simulink model "dc_servo_HighGainCommand"  (R2020b)
settings: Solver=ode5  StartTime=0.0  StopTime=.25  FixedStep=.00001  RelTol=1e-6  AbsTol=1e-6
values from neighbouring files (symbols this model uses):
  encoder = 2000    [dc_servo_HighGainCommand_data.m]    (also in dc_servo_speed_estimation_data.m)
  f = 4e-4    (= 0.0004)    [dc_servo_HighGainCommand_data.m]    (also in dc_servo_speed_estimation_data.m)
  imax = 5    [dc_servo_HighGainCommand_data.m]    (also in dc_servo_speed_estimation_data.m)
  integrator_saturation = 10000    [dc_servo_HighGainCommand_data.m]    (also in dc_servo_speed_estimation_data.m)
  J = 6.0e-5    (= 6e-05)    [dc_servo_HighGainCommand_data.m]    (also in dc_servo_speed_estimation_data.m)
  KI = k*k    (= 10000)    [dc_servo_HighGainCommand_data.m]    (also in dc_servo_speed_estimation_data.m)
  Kp = k    (= 100)    [dc_servo_HighGainCommand_data.m]    (also in dc_servo_speed_estimation_data.m = 200)
  KT = 0.07    [dc_servo_HighGainCommand_data.m]    (also in dc_servo_speed_estimation_data.m)
  L = 0.002    [dc_servo_HighGainCommand_data.m]    (also in dc_servo_speed_estimation_data.m)
  load_torque = 0    [dc_servo_HighGainCommand_data.m]    (also in dc_servo_speed_estimation_data.m)
  omega0 = 0    [dc_servo_HighGainCommand_data.m]    (also in dc_servo_speed_estimation_data.m)
  R = 2    [dc_servo_HighGainCommand_data.m]    (also in dc_servo_speed_estimation_data.m)
  theta0 = 0    [dc_servo_HighGainCommand_data.m]    (also in dc_servo_speed_estimation_data.m)
  vmax = 40    [dc_servo_HighGainCommand_data.m]    (also in dc_servo_speed_estimation_data.m)
libraries: simulink x1
settings Model: ExtModeTrigMode=oneshot  ExtModeArmWhenConnect=off  Creator=johnchiasson  LastModifiedBy=johnchiasson
settings DataIOCC: SaveFormat=Array  SignalLoggingSaveFormat=ModelDataLogs  SaveOutput=off  SaveTime=off  ReturnWorkspaceOutputs=off  SignalLoggingName=sigsOut
settings OptimizationCC: BlockReduction=off  BooleanDataType=off
settings DebuggingCC: SaveWithParameterizedLinksMsg=none  UnderspecifiedInitializationDetection=Classic  MergeDetectMultiDrivingBlocksExec=none  SignalResolutionControl=TryResolveAllWithWarning  MultiTaskDSMMsg=warning  MultiTaskCondExecSysMsg=none
settings HardwareCC: ProdBitPerPointer=32  ProdBitPerSizeT=32  ProdBitPerPtrDiffT=32  ProdLargestAtomicFloat=None  ProdIntDivRoundTo=Undefined  ProdEndianess=Unspecified  ProdWordSize=32  ProdHWDeviceType=32-bit Generic  TargetUnknown=on
settings ModelReferenceCC: PropagateSignalLabelsOutOfModel=off
settings GRTTargetCC: CombineOutputUpdateFcns=off  GRTInterface=on
settings ConfigComp: CovMetricSettings=dw  CovSaveCumulativeToWorkspaceVar=on  CovSaveSingleToWorkspaceVar=on

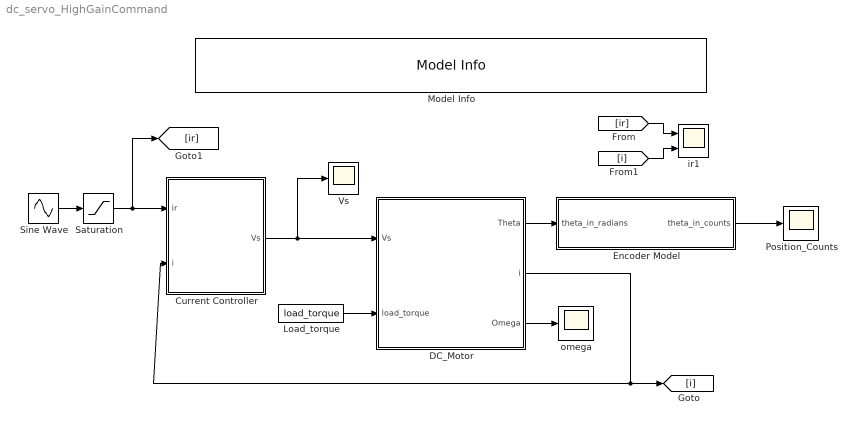
== system dc_servo_HighGainCommand ==
  Current Controller : Subsystem
  DC_Motor : Subsystem
  Encoder Model : Subsystem
  Load_torque : Constant  Value=load_torque
  Model Info : simulink/Model-Wide Utilities/Model Info  Frame=on  DisplayStringWithTags=High Gain Current Command  HorizontalTextAlignment=Center  LeftAlignmentValue=0.5
  Position_Counts : Scope
  Saturation : Saturate  UpperLimit=imax  LowerLimit=-imax
  Sine Wave : Sin  Amplitude=0.5  Frequency=2*pi/0.2  SampleTime=0
  Vs : Scope
  ir1 : Scope  NumInputPorts=2
  omega : Scope
  wires:
  Encoder Model/1(theta_in_counts) -> Position_Counts/1
  Sine Wave/1 -> Saturation/1
  DC_Motor/2(i) -> Current Controller/2(i), [i]
  Current Controller/1(Vs) -> DC_Motor/1(Vs), Vs/1
  DC_Motor/1(Theta) -> Encoder Model/1(theta_in_radians)
  Load_torque/1 -> DC_Motor/2(load_torque)
  DC_Motor/3(Omega) -> omega/1
  Saturation/1 -> [ir], Current Controller/1(ir)
  [ir] -> ir1/1
  [i] -> ir1/2

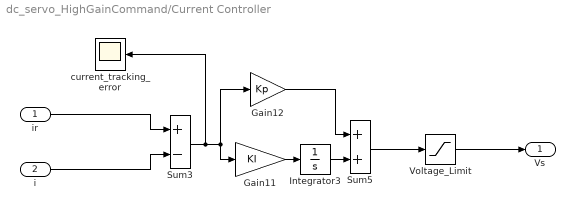
== system dc_servo_HighGainCommand/Current Controller ==
  ir : Inport
  i : Inport  Port=2
  Gain11 : Gain  Gain=KI  SaturateOnIntegerOverflow=on  OutDataTypeStr=Inherit: Same as input  ParamDataTypeStr=Inherit: Same as input
  Gain12 : Gain  Gain=Kp  SaturateOnIntegerOverflow=on  OutDataTypeStr=Inherit: Same as input  ParamDataTypeStr=Inherit: Same as input
  Integrator3 : Integrator
  Sum3 : Sum  Inputs=+-  InputSameDT=on  SaturateOnIntegerOverflow=on  OutDataTypeStr=Inherit: Same as first input
  Sum5 : Sum  InputSameDT=on  SaturateOnIntegerOverflow=on  OutDataTypeStr=Inherit: Same as first input
  Voltage_Limit : Saturate  UpperLimit=vmax  LowerLimit=-vmax
  current_tracking_error : Scope
  Vs : Outport
  wires:
  Sum3/1 -> current_tracking_error/1, Gain11/1, Gain12/1
  Gain12/1 -> Sum5/1
  Integrator3/1 -> Sum5/2
  Gain11/1 -> Integrator3/1
  Sum5/1 -> Voltage_Limit/1
  i/1 -> Sum3/2
  Voltage_Limit/1 -> Vs/1
  ir/1 -> Sum3/1

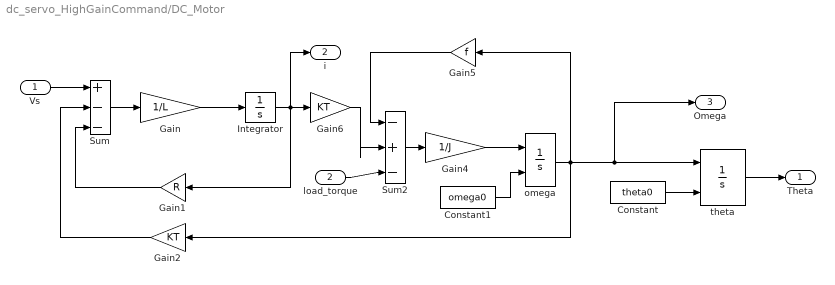
== system dc_servo_HighGainCommand/DC_Motor ==
  Vs : Inport
  load_torque : Inport  Port=2
  Constant : Constant  Value=theta0
  Constant1 : Constant  Value=omega0
  Gain : Gain  Gain=1/L  SaturateOnIntegerOverflow=on  OutDataTypeStr=Inherit: Same as input  ParamDataTypeStr=Inherit: Same as input
  Gain1 : Gain  Gain=R  SaturateOnIntegerOverflow=on  OutDataTypeStr=Inherit: Same as input  ParamDataTypeStr=Inherit: Same as input
  Gain2 : Gain  Gain=KT  SaturateOnIntegerOverflow=on  OutDataTypeStr=Inherit: Same as input  ParamDataTypeStr=Inherit: Same as input
  Gain4 : Gain  Gain=1/J  SaturateOnIntegerOverflow=on  OutDataTypeStr=Inherit: Same as input  ParamDataTypeStr=Inherit: Same as input
  Gain5 : Gain  Gain=f  SaturateOnIntegerOverflow=on  OutDataTypeStr=Inherit: Same as input  ParamDataTypeStr=Inherit: Same as input
  Gain6 : Gain  Gain=KT  SaturateOnIntegerOverflow=on  OutDataTypeStr=Inherit: Same as input  ParamDataTypeStr=Inherit: Same as input
  Integrator : Integrator  LimitOutput=on  UpperSaturationLimit=integrator_saturation  LowerSaturationLimit=-integrator_saturation
  Sum : Sum  Inputs=+--  InputSameDT=on  SaturateOnIntegerOverflow=on  OutDataTypeStr=Inherit: Same as first input
  Sum2 : Sum  Inputs=|-+-  InputSameDT=on  SaturateOnIntegerOverflow=on  OutDataTypeStr=Inherit: Same as first input
  omega : Integrator  InitialConditionSource=external  LimitOutput=on  UpperSaturationLimit=integrator_saturation  LowerSaturationLimit=-integrator_saturation
  theta : Integrator  InitialConditionSource=external  LimitOutput=on  UpperSaturationLimit=integrator_saturation  LowerSaturationLimit=-integrator_saturation
  Theta : Outport
  i : Outport  Port=2
  Omega : Outport  Port=3
  wires:
  Gain/1 -> Integrator/1
  Gain1/1 -> Sum/3
  Sum/1 -> Gain/1
  Vs/1 -> Sum/1
  Integrator/1 -> Gain1/1, Gain6/1, i/1
  Sum2/1 -> Gain4/1
  Gain6/1 -> Sum2/2
  Gain4/1 -> omega/1
  load_torque/1 -> Sum2/3
  omega/1 -> Gain5/1, theta/1, Omega/1, Gain2/1
  Gain5/1 -> Sum2/1
  theta/1 -> Theta/1
  Gain2/1 -> Sum/2
  Constant/1 -> theta/2
  Constant1/1 -> omega/2

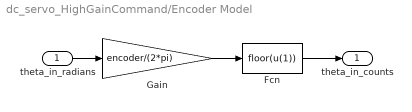
== system dc_servo_HighGainCommand/Encoder Model ==
  theta_in_radians : Inport
  Fcn : Fcn  Expr=floor(u(1))
  Gain : Gain  Gain=encoder/(2*pi)  SaturateOnIntegerOverflow=on  OutDataTypeStr=Inherit: Same as input  ParamDataTypeStr=Inherit: Same as input
  theta_in_counts : Outport
  wires:
  Gain/1 -> Fcn/1
  theta_in_radians/1 -> Gain/1
  Fcn/1 -> theta_in_counts/1
